simulink model "counter"  (R2016b)
settings: Solver=FixedStepDiscrete  StartTime=0.0  StopTime=1  RelTol=1e-3
libraries: simulink x2, slrtlib x1
settings Model: ExtModeTrigDuration=5  Creator=jays  LastModifiedBy=jays
settings OptimizationCC: MaxStackSize=64
settings DebuggingCC: ParameterTunabilityLossMsg=error
settings HardwareCC: ProdBitPerPointer=32  ProdBitPerSizeT=32  ProdBitPerPtrDiffT=32  ProdLargestAtomicInteger=Long  ProdLargestAtomicFloat=Double  ProdWordSize=32  ProdHWDeviceType=ARM Compatible->ARM Cortex
settings RTWCC: SystemTargetFile=ert.tlc  HardwareBoard=NXP FRDM-KL25Z  TLCOptions=-aInlineSetEventsForThisBaseRateFcn=TLC_FALSE -aSuppressMultiTaskScheduler=TLC_FALSE -aRateBasedStepFcn=1  TemplateMakefile=ert_default_tmf  Description=Embedded Coder  GenerateReport=on  Toolchain=GNU Tools for ARM Embedded Processors  IncludeHyperlinkInReport=on  LaunchReport=on  GenerateTraceInfo=on  GenerateTraceReport=on  GenerateTraceReportSl=on  GenerateTraceReportSf=on  GenerateTraceReportEml=on
settings CodeAppCC: ForceParamTrailComments=on  IgnoreCustomStorageClasses=off  OperatorAnnotations=on  SimulinkDataObjDesc=on  SFDataObjDesc=on  MATLABFcnDesc=on  InsertBlockDesc=on  MATLABSourceComments=on

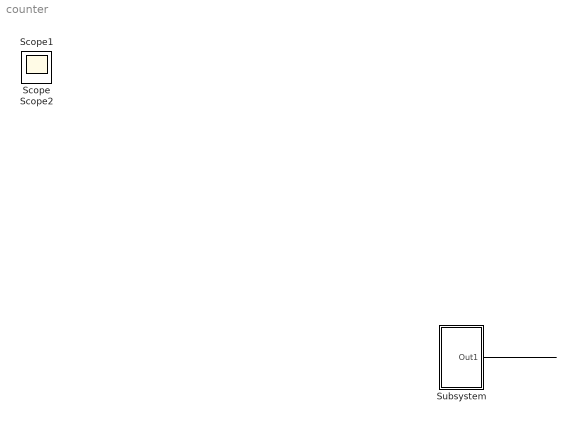
== system counter ==
  Subsystem : Subsystem
  Scope : Scope
  Scope1 : Scope
  Scope2 : Scope
  wires:
  Subsystem/1(Out1) -> ?

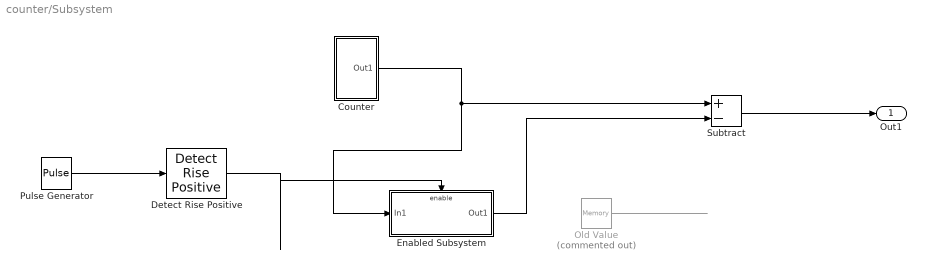
== system counter/Subsystem ==
  "Counter " : Subsystem
  Detect Rise Positive : simulink/Logic and Bit Operations/Detect Rise Positive  vinit=0  OutDataTypeStr=boolean
  Enabled Subsystem : Subsystem  TreatAsAtomicUnit=on
  Old Value : Memory  Commented=on
  Pulse Generator : DiscretePulseGenerator  PulseType=Time based  Period=0.02  PulseWidth=50
  Subtract : Sum  Inputs=+-
  Out1 : Outport
  wires:
  Old Value/1 -> ?
  Subtract/1 -> Out1/1
  "Counter "/1(Out1) -> Enabled Subsystem/1(In1), Subtract/1
  Enabled Subsystem/1(Out1) -> Subtract/2
  Detect Rise Positive/1 -> Enabled Subsystem/Enable
  Pulse Generator/1 -> Detect Rise Positive/1

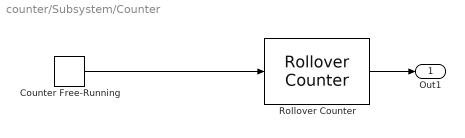
== system counter/Subsystem/Counter  ==
  Counter Free-Running : simulink/Sources/Counter Free-Running  NumBits=16  tsamp=0.001
  "Rollover Counter " : slrtlib/Incremental Encoder/Utilities/Rollover/Rollover Counter   InitialValue=0  RolloverThreshold=2^15
  Out1 : Outport
  wires:
  "Rollover Counter "/1 -> Out1/1
  Counter Free-Running/1 -> "Rollover Counter "/1

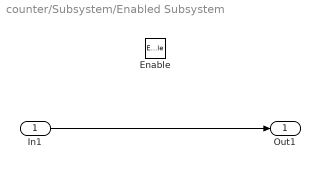
== system counter/Subsystem/Enabled Subsystem ==
  In1 : Inport
  Enable : EnablePort
  Out1 : Outport
  wires:
  In1/1 -> Out1/1
